simulink model "bola_levitador"  (Simulink 10.3)
settings: Solver=VariableStepAuto  StartTime=0.0  StopTime=25  RelTol=1e-3
model workspace (MAT data in the model file):
  a = Simulink.Parameter
  a.Value = 0.025
  a.DataType = 'auto'
  a.DocUnits = 'm'
  a.Dimensions = [1 1]
  alpha = Simulink.Parameter
  alpha.Value = 3.4154
  alpha.DataType = 'auto'
  alpha.Dimensions = [1 1]
  g = Simulink.Parameter
  g.Value = 9.81
  g.Description = 'Aceleração da gravidade'
  g.DataType = 'auto'
  g.DocUnits = 'm/s^2'
  g.Dimensions = [1 1]
  gama = Simulink.Parameter
  gama.Value = 0.1138
  gama.DataType = 'auto'
  gama.Dimensions = [1 1]
  k = Simulink.Parameter
  k.Value = 0.2
  k.DataType = 'auto'
  k.Dimensions = [1 1]
  ro_a = Simulink.Parameter
  ro_a.Value = 1.184
  ro_a.Description = 'Densidade do ar'
  ro_a.DataType = 'auto'
  ro_a.DocUnits = 'kg/m^3'
  ro_a.Dimensions = [1 1]
  ro_b = Simulink.Parameter
  ro_b.Value = 10.4
  ro_b.Description = 'Densidade esfera'
  ro_b.DataType = 'auto'
  ro_b.DocUnits = 'kg/m^3'
  ro_b.Dimensions = [1 1]
libraries: vrlib x4
settings Model: Creator=micha  LastModifiedBy=micha  EnablePacing=on  OrderedModelArguments=off
settings SolverCC: AlgebraicLoopSolver=Auto
settings DataIOCC: SaveFormat=Dataset  SignalLoggingSaveFormat=Dataset  ReturnWorkspaceOutputs=on
settings OptimizationCC: ExpressionDepthLimit=128  LifeSpan=auto
settings DebuggingCC: UnderspecifiedInitializationDetection=Simplified  MergeDetectMultiDrivingBlocksExec=error  FcnCallInpInsideContextMsg=error  StateNameClashWarn=none  SFUnexpectedBacktrackingDiag=error  SFNoUnconditionalDefaultTransitionDiag=error  SFExecutionAtInitializationDiag=warning  SFMachineParentedDataDiag=error  ArithmeticOperatorsInVariantConditions=error
settings HardwareCC: ProdBitPerPointer=64  ProdBitPerSizeT=64  ProdBitPerPtrDiffT=64  ProdLargestAtomicFloat=Float  ProdIntDivRoundTo=Zero  ProdEndianess=LittleEndian  ProdWordSize=64  ProdHWDeviceType=Intel->x86-64 (Windows64)
settings ModelReferenceCC: PropagateSignalLabelsOutOfModel=on
settings SFSimCC: SimUseLocalCustomCode=on  CustomCodeUndefinedFunction=FilterOut
settings RTWCC: RTWUseLocalCustomCode=on
settings CodeAppCC: StateflowObjectComments=off
settings GRTTargetCC: TargetLangStandard=C99 (ISO)  CombineOutputUpdateFcns=on  GRTInterface=off
settings ConfigComp: CovMetricSettings=dwe  CovSaveCumulativeToWorkspaceVar=off  CovSaveSingleToWorkspaceVar=off  CovExternalEMLEnable=on

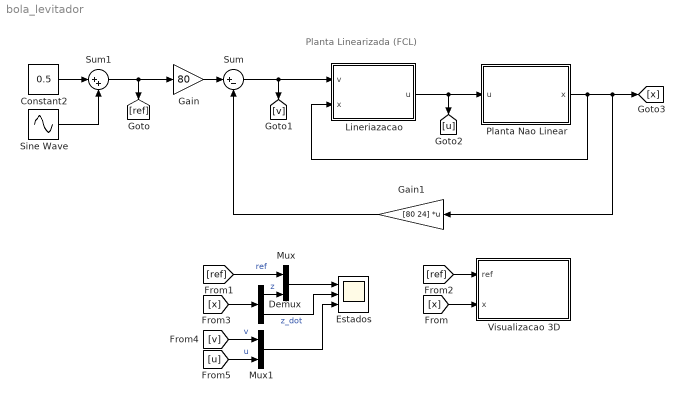
== system bola_levitador ==
  note: Planta Linearizada (FCL)
  Constant2 : Constant  Value=0.5
  Demux : Demux  Outputs=2
  Estados : Scope  NumInputPorts=3
  Gain : Gain  Gain=80
  Gain1 : Gain  Gain=[80 24]  Multiplication=Matrix(K*u)
  Lineriazacao : Subsystem
  Mux : Mux  Inputs=2
  Mux1 : Mux  Inputs=2
  Planta Nao Linear : Subsystem
  Sine Wave : Sin  Amplitude=0.05  SampleTime=0
  Sum : Sum  Inputs=|+-
  Sum1 : Sum  Inputs=|++
  Visualizacao 3D : Subsystem
  wires:
  Sum1/1 -> [ref], Gain/1
  Gain/1 -> Sum/1
  Lineriazacao/1(u) -> [u], Planta Nao Linear/1(u)
  Planta Nao Linear/1(x) -> Lineriazacao/2(x), Gain1/1, [x]
  Sum/1 -> [v], Lineriazacao/1(v)
  Gain1/1 -> Sum/2
  [ref] -> Visualizacao 3D/1(ref)
  [x] -> Visualizacao 3D/2(x)
  [x] -> Demux/1
  [v] -> Mux1/1  "v"
  [u] -> Mux1/2  "u"
  Mux/1 -> Estados/1
  [ref] -> Mux/1  "ref"
  Demux/1 -> Mux/2  "z"
  Demux/2 -> Estados/2  "z_dot"
  Sine Wave/1 -> Sum1/2
  Constant2/1 -> Sum1/1
  Mux1/1 -> Estados/3

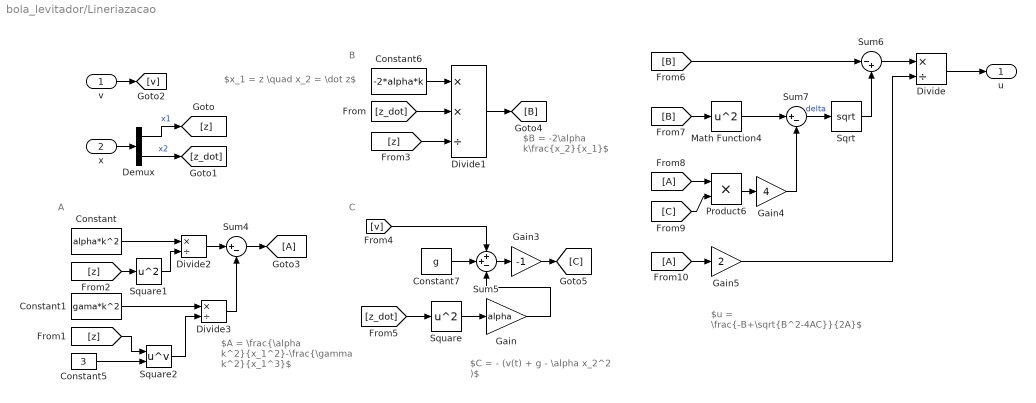
== system bola_levitador/Lineriazacao ==
  note: $C = - (v(t) + g - \alpha x_2^2 )$
  note: $B = -2\alpha k\frac{x_2}{x_1}$
  note: $x_1 = z \quad x_2 = \dot z$
  note: $A = \frac{\alpha k^2}{x_1^2}-\frac{\gamma k^2}{x_1^3}$
  note: $u = \frac{-B+\sqrt{B^2-4AC}}{2A}$
  note: A
  note: B
  note: C
  v : Inport
  x : Inport  Port=2
  Constant : Constant  Value=alpha*k^2
  Constant1 : Constant  Value=gama*k^2
  Constant5 : Constant  Value=3
  Constant6 : Constant  Value=-2*alpha*k
  Constant7 : Constant  Value=g
  Demux : Demux  Outputs=2
  Divide : Product  Inputs=*/
  Divide1 : Product  Inputs=**/
  Divide2 : Product  Inputs=*/
  Divide3 : Product  Inputs=*/
  Gain : Gain  Gain=alpha
  Gain3 : Gain  Gain=-1
  Gain4 : Gain  Gain=4
  Gain5 : Gain  Gain=2
  Math Function4 : Math  Operator=square  SaturateOnIntegerOverflow=on
  Product6 : Product
  Sqrt : Sqrt  SaturateOnIntegerOverflow=on
  Square : Math  Operator=square  SaturateOnIntegerOverflow=on
  Square1 : Math  Operator=square  SaturateOnIntegerOverflow=on
  Square2 : Math  Operator=pow  SaturateOnIntegerOverflow=on
  Sum4 : Sum  Inputs=|+-
  Sum5 : Sum  Inputs=++-
  Sum6 : Sum  Inputs=|-+
  Sum7 : Sum  Inputs=|+-
  u : Outport
  wires:
  [B] -> Sum6/1
  Gain/1 -> Sum5/3
  Sum6/1 -> Divide/1
  [A] -> Gain5/1
  Constant7/1 -> Sum5/2
  Gain3/1 -> [C]
  Sum7/1 -> Sqrt/1  "delta"
  Sum4/1 -> [A]
  Divide/1 -> u/1
  Gain5/1 -> Divide/2
  Sum5/1 -> Gain3/1
  [B] -> Math Function4/1
  [A] -> Product6/1
  Gain4/1 -> Sum7/2
  Math Function4/1 -> Sum7/1
  Product6/1 -> Gain4/1
  Sqrt/1 -> Sum6/2
  [C] -> Product6/2
  x/1 -> Demux/1
  Demux/2 -> [z_dot]  "x2"
  v/1 -> [v]
  [v] -> Sum5/1
  Constant6/1 -> Divide1/1
  [z_dot] -> Divide1/2
  [z] -> Divide1/3
  Divide1/1 -> [B]
  [z_dot] -> Square/1
  Square/1 -> Gain/1
  [z] -> Square1/1
  Divide3/1 -> Sum4/2
  Constant5/1 -> Square2/2
  [z] -> Square2/1
  Demux/1 -> [z]  "x1"
  Divide2/1 -> Sum4/1
  Square1/1 -> Divide2/2
  Constant/1 -> Divide2/1
  Square2/1 -> Divide3/2
  Constant1/1 -> Divide3/1

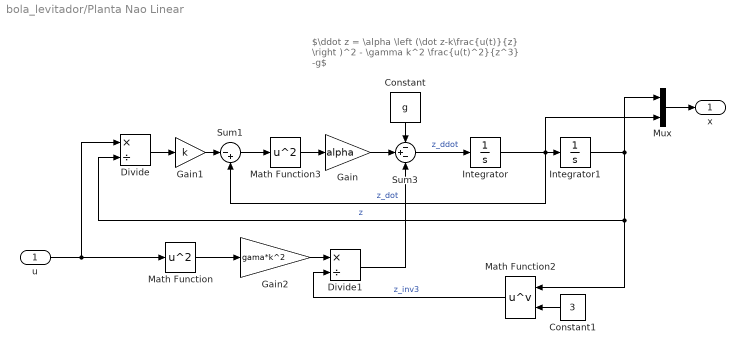
== system bola_levitador/Planta Nao Linear ==
  note: $\ddot z = \alpha \left (\dot z-k\frac{u(t)}{z} \right )^2 - \gamma k^2 \frac{u(t)^2}{z^3} -g$
  u : Inport
  Constant : Constant  Value=g
  Constant1 : Constant  Value=3
  Divide : Product  Inputs=*/
  Divide1 : Product  Inputs=*/
  Gain : Gain  Gain=alpha
  Gain1 : Gain  Gain=k
  Gain2 : Gain  Gain=gama*k^2
  Integrator : Integrator
  Integrator1 : Integrator  InitialCondition=0.035
  Math Function : Math  Operator=square  SaturateOnIntegerOverflow=on
  Math Function2 : Math  Operator=pow  SaturateOnIntegerOverflow=on
  Math Function3 : Math  Operator=square  SaturateOnIntegerOverflow=on
  Mux : Mux  Inputs=2
  Sum1 : Sum  Inputs=|-+
  Sum3 : Sum  Inputs=-+-
  x : Outport
  wires:
  Math Function3/1 -> Gain/1
  Sum1/1 -> Math Function3/1
  Math Function2/1 -> Divide1/2  "z_inv3"
  Gain2/1 -> Divide1/1
  Constant1/1 -> Math Function2/2
  Math Function/1 -> Gain2/1
  Integrator1/1 -> Mux/1, Divide/2, Math Function2/1  "z"
  Integrator/1 -> Mux/2, Integrator1/1, Sum1/2  "z_dot"
  Sum3/1 -> Integrator/1  "z_ddot"
  Divide/1 -> Gain1/1
  u/1 -> Divide/1, Math Function/1
  Constant/1 -> Sum3/1
  Gain/1 -> Sum3/2
  Gain1/1 -> Sum1/1
  Divide1/1 -> Sum3/3
  Mux/1 -> x/1

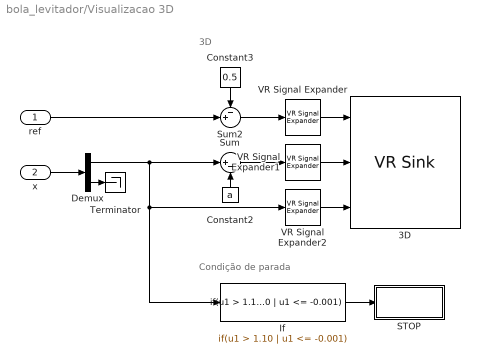
== system bola_levitador/Visualizacao 3D ==
  note: 3D
  note: Condição de parada
  ref : Inport
  x : Inport  Port=2
  3D : vrlib/VR Sink  InstantiateOnLoad=on  SampleTime=0.05  ViewEnable=on  RemoteChange=off  RemoteView=off  FieldsWritten=Indicador.translation.3.1.1.double#Esfera.translation.3.1.1.double#Zoom.position.3.1.1.double  WorldFileName=modelo3d.x3d  AutoView=on  VideoDimensions=[]  AllowVariableSize=off
  Constant2 : Constant  Value=a
  Constant3 : Constant  Value=0.5
  Demux : Demux  Outputs=2
  If : If  IfExpression=u1 > 1.10 | u1 <= -0.001  ShowElse=off
  STOP : Subsystem  TreatAsAtomicUnit=on
  Sum : Sum  Inputs=|+-
  Sum2 : Sum  Inputs=-+|
  Terminator : Terminator
  VR Signal Expander : vrlib/VR Signal Expander  outwidth=3  outidx=2
  VR Signal Expander1 : vrlib/VR Signal Expander  outwidth=3  outidx=2
  VR Signal Expander2 : vrlib/VR Signal Expander  outwidth=3  outidx=2
  wires:
  VR Signal Expander1/1 -> 3D/2
  Constant3/1 -> Sum2/1
  Sum/1 -> VR Signal Expander1/1
  Sum2/1 -> VR Signal Expander/1
  Constant2/1 -> Sum/2
  If/1 -> STOP/Action
  VR Signal Expander/1 -> 3D/1
  ref/1 -> Sum2/2
  VR Signal Expander2/1 -> 3D/3
  x/1 -> Demux/1
  Demux/1 -> If/1, VR Signal Expander2/1, Sum/1
  Demux/2 -> Terminator/1

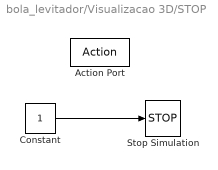
== system bola_levitador/Visualizacao 3D/STOP ==
  Action Port : ActionPort  ActionPortLabel=if(u1 > 1.10 | u1 <= -0.001)
  Constant : Constant
  Stop Simulation : Stop
  wires:
  Constant/1 -> Stop Simulation/1
